simulink model "exercitiul3colocviuTS2"  (R2021b)
settings: Solver=VariableStepAuto  StartTime=0.0  StopTime=10.0  RelTol=1e-3

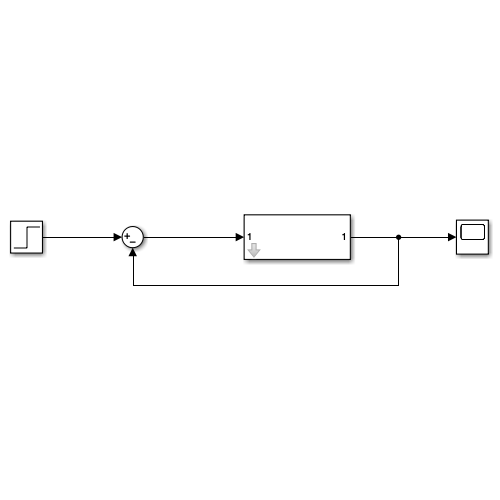
[thumbnail: Simulink's stored preview of the top-level diagram]
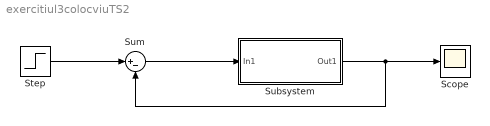
== system exercitiul3colocviuTS2 ==
  Scope : Scope
  Step : Step  SampleTime=0
  Subsystem : Subsystem  mask{a1=6}
      mask init:
      | if str2num(get_param(gcb, 'a1'))<5
      |           error('nu se afla in interval')
      | end
      | if str2num(get_param(gcb, 'a1'))>7
      |           error('nu se afla in interval')
      | end
  Sum : Sum  Inputs=|+-
  wires:
  Sum/1 -> Subsystem/1(In1)
  Step/1 -> Sum/1
  Subsystem/1(Out1) -> Sum/2, Scope/1

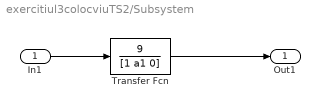
== system exercitiul3colocviuTS2/Subsystem ==
  In1 : Inport
  Transfer Fcn : TransferFcn  Numerator=[9]  Denominator=[1 a1 0]
  Out1 : Outport
  wires:
  In1/1 -> Transfer Fcn/1
  Transfer Fcn/1 -> Out1/1
